simulink model "BANSHEE"  (Simulink 8.7)
settings: Solver=ode1  StartTime=0.0  StopTime=inf  FixedStep=Ts  MaxStep=1e-3  RelTol=1e-3
PostLoadFcn:
  | BANSHEE_init;
InitFcn:
  | BANSHEE_init;
values from neighbouring files (symbols this model uses):
  Ts = 100E-6    (= 0.0001)    [BANSHEE_init.m]
undefined symbols (not defined in the file or in its folder): Acid, Banshee_HWCtrl_IOs, Banshee_SEL751_Woodward_lib, DMS_slave_lib, DMSCommands, F1, F2, F3, fdesignblkfcn, Feeder1_lib, Feeder2_lib, Feeder3_lib, gcbh, generic_ethernet_cb, Lead, Left, relay_housing_lib, SM_UtilityService, SS_F1_RELAY_HOUSING, SS_F2_RELAY_HOUSING, SS_F3_RELAY_HOUSING, SS_Feeder1, SS_Feeder2, SS_Feeder3, SUBSTATION, TestSeq_slave_lib, TestSequenceCommands, type, utility_service_lib, V
libraries: powerlib x108, cables_lib x61, breaker_lib x53, rtio_generic_modbus x50, relay_modbus_lib x45, rtio_opalrt_op5142ex1 x37, transformer_lib x29, rteventslib x28, Load_lib x25, simulink x24, rtlab x20, ssn_lib x19
(part 5 of 9)

== system BANSHEE/SS_F3_RELAY_HOUSING/Banshee UDP Data - Formatted Packets ==
  note: The Number of data to send should match the size of Mux-to-Ethernet
  note: Copyright (c) 2016 Massachusetts Institute of Technology
      | Permission is hereby granted, free of charge, to any person obtaining a copy of this software and associated documentation files (the "Software"), to deal
      | in the Software without restriction, including without limitation the rights to use, copy, modify, merge, publish, distribute, sublicense, and/or sell copies of the
      | Software, and to permit persons to whom the Software is furnished to do so, subject to the following conditions:
      |
      | THE SOFTWARE IS PROVIDED "AS IS", WITHOUT WARRANTY OF ANY KIND, EXPRESS OR IMPLIED, INCLUDING BUT NOT LIMITED TO THE
      | WARRANTIES OF MERCHANTABILITY, FITNESS FOR A PARTICULAR PURPOSE AND NONINFRINGEMENT. IN NO EVENT SHALL THE AUTHORS
      | OR COPYRIGHT HOLDERS BE LIABLE FOR ANY CLAIM, DAMAGES OR OTHER LIABILITY, WHETHER IN AN ACTION OF CONTRACT, TORT OR
      | OTHERWISE, ARISING FROM, OUT OF OR IN CONNECTION WITH THE SOFTWARE OR THE USE OR OTHER DEALINGS IN THE SOFTWARE
  Time Stamp : Inport
  Waveforms : Inport  Port=2  PortDimensions=3
  Relay Data : Inport  Port=3
  BESS Data : Inport  Port=4
  Diesel Gensets Data : Inport  Port=5
  NGCHP Gensets Data : Inport  Port=6
  Motors Data : Inport  Port=7
  PV Data : Inport  Port=8
  Power Factor Data : Inport  Port=9
  Miscellaneous Data : Inport  Port=10
  " # of motors" : Constant  Value=NumOfMotors  OutDataTypeStr=double
  " # of motors1" : Constant  Value=NumOfMiscellaneousDataScales  OutDataTypeStr=double
  # of Batteries : Constant  Value=NumOfBatteries  OutDataTypeStr=double
  # of PVs : Constant  Value=NumOfPVs  OutDataTypeStr=double
  # of PVs1 : Constant  Value=NumOfMiscellaneousDataSignalsScales  OutDataTypeStr=double
  # of PVs2 : Constant  Value=NumOfPF  OutDataTypeStr=double
  # of Relays : Constant  Value=NumOfRelays  OutDataTypeStr=double
  # of Waveform s : Constant  Value=NumOfWaveforms  OutDataTypeStr=double
  # of gensets : Constant  Value=NumOfDieselGensets  OutDataTypeStr=double
  # of gensets1 : Constant  Value=NumOfNGCHPGensets  OutDataTypeStr=double
  Cast uint16 : MATLAB Function  TreatAsAtomicUnit=on
  Checksum : Sum  Inputs=+
  Data Type Conversion : DataTypeConversion
  Data Type Conversion1 : DataTypeConversion  OutDataTypeStr=uint32  ConvertRealWorld=Stored Integer (SI)  RndMeth=Nearest
  Ethernet communication interface : Subsystem  mask(AsyncEthernet){ctrl_id=1, nbr_to_remote_endpoint=375, type_to_remote_endpoint=INT32, offset_to_remote_endpoint=0, swap_tx=off, nbr_from_remote_endpoint=4, type_from_remote_endpoint=DOUBLE, offset_from_remote_endpoint=0, swap_rx=off, exe_name='AsyncEthernet', nic_name='eth0', protocol=UDP, tcp_mode=Server, port=7200, remote_ip='255.255.255.255'}
      mask prompts: ctrl_id "Controller ID"; nbr_to_remote_endpoint "Number of data to send"; type_to_remote_endpoint "Type of data to send"; offset_to_remote_endpoint "Byte offset of transmission buffer"; swap_tx "Swap data endianness before transmission"; nbr_from_remote_endpoint "Number of data expected to be received"; type_from_remote_endpoint "Type of data expected to be received"; offset_from_remote_endpoint "Byte offset of reception buffer"; swap_rx "Swap data endianness after reception"; exe_name "Executable name"; nic_name "Network interface name"; tcp_mode "TCP mode"; port "Port number"; remote_ip "Remote IP address"
      mask help: This block is used as a communication interface to send data to a remote dedevice and receive data from it.
      mask Help: eval('rtlab_io_help(''Generic/Ethernet/Ethernet_interface.htm'');');
      mask Callback ctrl_id:
      | var = get_param(gcb,'ctrl_id');
      | set_param([gcb '/AsyncEthernetCtrl'],'ctrl_id',var)
      mask Callback nbr_to_remote_endpoint:
      | var = get_param(gcb,'nbr_to_remote_endpoint');
      | set_param([gcb '/AsyncEthernetCtrl'],'nbr_to_remote_endpoint',var)
      mask TypeOptions type_to_remote_endpoint: UINT8 | INT8 | UINT16 | INT16 | UINT32 | INT32 | FLOAT | DOUBLE
      mask Callback type_to_remote_endpoint:
      | var = get_param(gcb,'type_to_remote_endpoint');
      | set_param([gcb '/AsyncEthernetCtrl'],'type_to_remote_endpoint',var)
      mask Callback offset_to_remote_endpoint:
      | var = get_param(gcb,'offset_to_remote_endpoint');
      | set_param([gcb '/AsyncEthernetCtrl'],'offset_to_remote_endpoint',var)
      mask Callback swap_tx:
      | var = get_param(gcb,'swap_tx');
      | set_param([gcb '/AsyncEthernetCtrl'],'swap_tx',var)
      mask Callback nbr_from_remote_endpoint:
      | var = get_param(gcb,'nbr_from_remote_endpoint');
      | set_param([gcb '/AsyncEthernetCtrl'],'nbr_from_remote_endpoint',var)
      mask TypeOptions type_from_remote_endpoint: UINT8 | INT8 | UINT16 | INT16 | UINT32 | INT32 | FLOAT | DOUBLE
      mask Callback type_from_remote_endpoint:
      | var = get_param(gcb,'type_from_remote_endpoint');
      | set_param([gcb '/AsyncEthernetCtrl'],'type_from_remote_endpoint',var)
      mask Callback offset_from_remote_endpoint:
      | var = get_param(gcb,'offset_from_remote_endpoint');
      | set_param([gcb '/AsyncEthernetCtrl'],'offset_from_remote_endpoint',var)
      mask Callback swap_rx:
      | var = get_param(gcb,'swap_rx');
      | set_param([gcb '/AsyncEthernetCtrl'],'swap_rx',var)
      mask Callback exe_name:
      | str = get_param(gcb,'exe_name');
      | 
      | if exist('str','var')
      |     str = eval(str);
      | end
      | 
      | set_param([gcb '/AsyncEthernetCtrl'],'exe_name',str)
      mask Callback nic_name:
      | str = get_param(gcb,'nic_name');
      | 
      | if exist('str','var')
      |     str = eval(str);
      | end
      | 
      | set_param([gcb '/AsyncEthernetCtrl'],'nic_name',str)
      mask TypeOptions protocol: UDP | TCP
      mask Callback protocol: generic_ethernet_cb('protocol')
      mask TypeOptions tcp_mode: Client | Server
      mask Callback tcp_mode: generic_ethernet_cb('tcp_mode')
      mask Callback port:
      | var = get_param(gcb,'port');
      | set_param([gcb '/AsyncEthernetCtrl'],'port',var)
      mask Callback remote_ip:
      | str = get_param(gcb,'remote_ip');
      | 
      | if exist('str','var')
      |     str = eval(str);
      | end
      | 
      | set_param([gcb '/AsyncEthernetCtrl'],'remote_ip',str)
  Mux-to-Ethernet : Mux  Inputs=2
  Mux1 : Mux  Inputs=14
  Mux8 : Mux  Inputs=10
  Profile ID : Constant  Value=ProfileID  OutDataTypeStr=double
  Pulse input : DiscretePulseGenerator  PulseType=Time based  Period=1/5  PulseWidth=1/20
  Start Word 0xAFAF : Constant  Value=44975  OutDataTypeStr=double
  Stop Word 0x5555 : Constant  Value=21845  OutDataTypeStr=double
  wires:
  Start Word 0xAFAF/1 -> Mux1/1
  Pulse input/1 -> Data Type Conversion/1
  Data Type Conversion/1 -> Ethernet communication interface/1(Data trigger)
  Mux1/1 -> Mux8/1
  Checksum/1 -> Cast uint16/1(u)
  Cast uint16/1(y) -> Mux-to-Ethernet/2
  Mux-to-Ethernet/1 -> Ethernet communication interface/2(Data to send)
  Data Type Conversion1/1 -> Checksum/1
  Waveforms/1 -> Mux1/14
  BESS Data/1 -> Mux8/3
  Diesel Gensets Data/1 -> Mux8/4
  Relay Data/1 -> Mux8/2
  Mux8/1 -> Mux-to-Ethernet/1, Data Type Conversion1/1
  Stop Word 0x5555/1 -> Mux8/10
  NGCHP Gensets Data/1 -> Mux8/5
  Miscellaneous Data/1 -> Mux8/9
  Power Factor Data/1 -> Mux8/8
  PV Data/1 -> Mux8/7
  Motors Data/1 -> Mux8/6
  Time Stamp/1 -> Mux1/3
  # of PVs1/1 -> Mux1/13
  " # of motors1"/1 -> Mux1/12
  # of gensets1/1 -> Mux1/8
  # of gensets/1 -> Mux1/7
  # of Waveform s/1 -> Mux1/4
  " # of motors"/1 -> Mux1/9
  # of Batteries/1 -> Mux1/6
  # of PVs/1 -> Mux1/10
  # of PVs2/1 -> Mux1/11
  # of Relays/1 -> Mux1/5
  Profile ID/1 -> Mux1/2

== system BANSHEE/SS_F3_RELAY_HOUSING/DMSCommands ==
  note: Copyright (c) 2016 Massachusetts Institute of Technology
      | Permission is hereby granted, free of charge, to any person obtaining a copy of this software and associated documentation files (the "Software"), to deal
      | in the Software without restriction, including without limitation the rights to use, copy, modify, merge, publish, distribute, sublicense, and/or sell copies of the
      | Software, and to permit persons to whom the Software is furnished to do so, subject to the following conditions:
      |
      | THE SOFTWARE IS PROVIDED "AS IS", WITHOUT WARRANTY OF ANY KIND, EXPRESS OR IMPLIED, INCLUDING BUT NOT LIMITED TO THE
      | WARRANTIES OF MERCHANTABILITY, FITNESS FOR A PARTICULAR PURPOSE AND NONINFRINGEMENT. IN NO EVENT SHALL THE AUTHORS
      | OR COPYRIGHT HOLDERS BE LIABLE FOR ANY CLAIM, DAMAGES OR OTHER LIABILITY, WHETHER IN AN ACTION OF CONTRACT, TORT OR
      | OTHERWISE, ARISING FROM, OUT OF OR IN CONNECTION WITH THE SOFTWARE OR THE USE OR OTHER DEALINGS IN THE SOFTWARE
  Add : Sum
  Bus Creator : BusCreator  Inputs=11
  Demux : Demux  Outputs=14
  Gain : Gain  Gain=2^16
  Modbus device : rtio_generic_modbus/Modbus device  conf_name=DMS_cfg.opal  conf_name_mask=DMS_cfg.xls  sample_time=Ts
  Terminator : Terminator
  Terminator1 : Terminator
  DMS Data : Outport
  wires:
  Demux/11 -> Bus Creator/8  "VAR Value"
  Demux/10 -> Bus Creator/7  "VAR Active"
  Demux/9 -> Bus Creator/6  "PF Value"
  Demux/8 -> Bus Creator/5  "PF Active"
  Demux/3 -> Terminator1/1  "Fault1"
  Demux/4 -> Terminator/1  "Fault2"
  Demux/7 -> Bus Creator/4  "Limit Value"
  Demux/6 -> Bus Creator/3  "Limit Active"
  Demux/5 -> Bus Creator/2  "Disconnect"
  Modbus device/1 -> Demux/1
  Gain/1 -> Add/2
  Demux/2 -> Gain/1
  Demux/1 -> Add/1
  Add/1 -> Bus Creator/1  "TimeStamp"
  Bus Creator/1 -> DMS Data/1
  Demux/13 -> Bus Creator/10  "MGC_start"
  Demux/12 -> Bus Creator/9  "AutoSync_available"
  Demux/14 -> Bus Creator/11  "BlackStart"

== system BANSHEE/SS_F3_RELAY_HOUSING/SEL751-UDP ==
  note: Order of signals:
      | F3_PCC
      | F2_PCC
      | F1_PCC
      | F3_GCB (NG/CHP)
      | F1_GCB (DIESEL)
  note: % Copyright (c) 2016 Massachusetts Institute of Technology
      | % Permission is hereby granted, free of charge, to any person obtaining a copy of this
      | % software and associated documentation files (the "Software"), to deal in the Software
      | % without restriction, including without limitation the rights to use, copy, modify,
      | % merge, publish, distribute, sublicense, and/or sell copies of the Software, and to
      | % permit persons to whom the Software is furnished to do so, subject to the following
      | % conditions:
      | %
      | %
      | % The above copyright notice and this permission notice shall be included in
      | % all copies or substantial portions of the Software.
      | %
      | % THE SOFTWARE IS PROVIDED "AS IS", WITHOUT WARRANTY OF ANY KIND, EXPRESS OR IMPLIED,
      | % INCLUDING BUT NOT LIMITED TO THE WARRANTIES OF MERCHANTABILITY, FITNESS FOR A
      | % PARTICULAR PURPOSE AND NONINFRINGEMENT. IN NO EVENT SHALL THE AUTHORS OR COPYRIGHT
      | % HOLDERS BE LIABLE FOR ANY CLAIM, DAMAGES OR OTHER LIABILITY, WHETHER IN AN ACTION
      | % OF CONTRACT, TORT OR OTHERWISE, ARISING FROM, OUT OF OR IN CONNECTION WITH THE
      | % SOFTWARE OR THE USE OR OTHER DEALINGS IN THE SOFTWARE.
      | %
      | %
      | %%
  F3_MS : Inport
  F2_MS : Inport  Port=2
  F1_MS : Inport  Port=3
  Bus Creator : BusCreator  Inputs=5
  Bus Selector : BusSelector  OutputSignals=CB_DATA.F3_PCC
  Bus Selector3 : BusSelector  OutputSignals=CB_DATA.F2_PCC
  Bus Selector5 : BusSelector  OutputSignals=CB_DATA.F1_PCC
  PQFV : PQFV_lib/PQFV  VRMSLL=13800  Ts=Ts
  PQFV1 : PQFV_lib/PQFV  VRMSLL=13800  Ts=Ts
  PQFV2 : PQFV_lib/PQFV  VRMSLL=13800  Ts=Ts
  PQVF_out : Outport
  wires:
  Bus Selector/1 -> PQFV/1  "<F3_PCC>"
  Bus Selector3/1 -> PQFV1/1  "<F2_PCC>"
  F2_MS/1 -> Bus Selector3/1
  Bus Selector5/1 -> PQFV2/1  "<F1_PCC>"
  PQFV1/1 -> Bus Creator/2  "F2_PCC"
  PQFV/1 -> Bus Creator/1  "F3_PCC"
  PQFV2/1 -> Bus Creator/3  "F1_PCC"
  F3_MS/1 -> Bus Creator/4, Bus Selector/1  "F3_MS"
  F1_MS/1 -> Bus Creator/5, Bus Selector5/1  "F1_MS"
  Bus Creator/1 -> PQVF_out/1

== system BANSHEE/SS_Feeder1/fault_signal ==
  fault_ts : Inport
  fault_sc : Inport  Port=2
  Bus Selector26 : BusSelector  OutputSignals=fault_location_2
  Bus Selector28 : BusSelector  OutputSignals=fault_location_2
  Logical Operator : Logic  Operator=OR  AllPortsSameDT=off  OutDataTypeStr=boolean
  o : Outport
  wires:
  fault_sc/1 -> Bus Selector26/1
  Bus Selector26/1 -> Logical Operator/2  "<fault_location_2>"
  fault_ts/1 -> Bus Selector28/1
  Logical Operator/1 -> o/1
  Bus Selector28/1 -> Logical Operator/1  "<fault_location_2>"

== system BANSHEE/SS_Feeder1/fault_signal1 ==
  fault_ts : Inport
  fault_sc : Inport  Port=2
  Bus Selector26 : BusSelector  OutputSignals=fault_location_3
  Bus Selector28 : BusSelector  OutputSignals=fault_location_3
  Logical Operator : Logic  Operator=OR  AllPortsSameDT=off  OutDataTypeStr=boolean
  o : Outport
  wires:
  fault_sc/1 -> Bus Selector26/1
  Bus Selector26/1 -> Logical Operator/2  "<fault_location_3>"
  fault_ts/1 -> Bus Selector28/1
  Logical Operator/1 -> o/1
  Bus Selector28/1 -> Logical Operator/1  "<fault_location_3>"

== system BANSHEE/SS_Feeder2/fault_signal ==
  fault_ts : Inport
  fault_sc : Inport  Port=2
  Bus Selector26 : BusSelector  OutputSignals=fault_location_5
  Bus Selector28 : BusSelector  OutputSignals=fault_location_5
  Logical Operator : Logic  Operator=OR  AllPortsSameDT=off  OutDataTypeStr=boolean
  o : Outport
  wires:
  fault_sc/1 -> Bus Selector26/1
  Bus Selector26/1 -> Logical Operator/2  "<fault_location_5>"
  fault_ts/1 -> Bus Selector28/1
  Logical Operator/1 -> o/1
  Bus Selector28/1 -> Logical Operator/1  "<fault_location_5>"

== system BANSHEE/SS_Feeder2/fault_signal1 ==
  fault_ts : Inport
  fault_sc : Inport  Port=2
  Bus Selector26 : BusSelector  OutputSignals=fault_location_1
  Bus Selector28 : BusSelector  OutputSignals=fault_location_1
  Logical Operator : Logic  Operator=OR  AllPortsSameDT=off  OutDataTypeStr=boolean
  o : Outport
  wires:
  fault_sc/1 -> Bus Selector26/1
  Bus Selector26/1 -> Logical Operator/2  "<fault_location_1>"
  fault_ts/1 -> Bus Selector28/1
  Logical Operator/1 -> o/1
  Bus Selector28/1 -> Logical Operator/1  "<fault_location_1>"

== system BANSHEE/SS_Feeder3/HWController_3.5MVA_NGCHP ==
  note: Copyright (c) 2016 Massachusetts Institute of Technology
      | Permission is hereby granted, free of charge, to any person obtaining a copy of this software and associated documentation files (the "Software"), to deal
      | in the Software without restriction, including without limitation the rights to use, copy, modify, merge, publish, distribute, sublicense, and/or sell copies of the
      | Software, and to permit persons to whom the Software is furnished to do so, subject to the following conditions:
      |
      | THE SOFTWARE IS PROVIDED "AS IS", WITHOUT WARRANTY OF ANY KIND, EXPRESS OR IMPLIED, INCLUDING BUT NOT LIMITED TO THE
      | WARRANTIES OF MERCHANTABILITY, FITNESS FOR A PARTICULAR PURPOSE AND NONINFRINGEMENT. IN NO EVENT SHALL THE AUTHORS
      | OR COPYRIGHT HOLDERS BE LIABLE FOR ANY CLAIM, DAMAGES OR OTHER LIABILITY, WHETHER IN AN ACTION OF CONTRACT, TORT OR
      | OTHERWISE, ARISING FROM, OUT OF OR IN CONNECTION WITH THE SOFTWARE OR THE USE OR OTHER DEALINGS IN THE SOFTWARE
  Heat Load MBtu/hrs : Inport
  In2 : Inport  Port=2
  HWControllerBias : Inport  Port=3
  Bus Creator2 : BusCreator  Inputs=6
  Bus Selector6 : BusSelector  OutputSignals=Heat Recovered; MBtu/hr
  Bus Selector7 : BusSelector  OutputSignals=TempActual,HeatFromBoiler MBtu/hr,CHPHeatContribution MBtu/hr,Thermal data.Heat Recovered; MBtu/hr,Thermal data.CO2 lbm/hr,Boiler_Nm^3/hr ,Boiler lbm/hr CO2
  CHPThermalModel : CHP_Model_lib/CHPThermalModel  SIM_HIL=SIM_HIL
  Demux : Demux  Outputs=2
  HWController_NG_Generator : HWController_NGCHP_Genset_3p5MVA_lib/HWController_NG_Generator
  Modbus device : rtio_generic_modbus/Modbus device  conf_name=CHP_slave_cfg.opal  conf_name_mask=CHP_slave_cfg.xls  sample_time=Ts
  Mux1 : Mux  Inputs=7
  A : PMIOPort  Tag=A  Port=1  Side=Right
      settings: AttributesFormatString=A
  B : PMIOPort  Port=2  Side=Right
  C : PMIOPort  Port=3  Side=Right
  Out1 : Outport
  Generator Data : Outport  Port=2
  GCB Control : Outport  Port=3
  wires:
  Bus Selector7/6 -> Mux1/6  "<Boiler_Nm^3/hr >"
  Bus Selector7/7 -> Mux1/7  "<Boiler lbm/hr CO2 >"
  CHPThermalModel/5 -> Bus Creator2/6
  CHPThermalModel/4 -> Bus Creator2/5
  HWControllerBias/1 -> HWController_NG_Generator/1
  HWController_NG_Generator/3 -> [HeatRec_MBtuhr]  "Thermal data"
  Bus Selector7/3 -> Mux1/3  "<CHPHeatContribution MBtu/hr>"
  CHPThermalModel/1 -> Bus Creator2/2  "TempActual"
  Demux/2 -> CHPThermalModel/4
  CHPThermalModel/2 -> Bus Creator2/3
  Bus Selector7/2 -> Mux1/2  "<HeatFromBoiler MBtu/hr>"
  Bus Selector7/5 -> Mux1/5  "<CO2 lbm/hr>"
  Bus Selector7/4 -> Mux1/4  "<Heat Recovered; MBtu/hr>"
  Bus Selector7/1 -> Mux1/1  "<TempActual>"
  Heat Load MBtu/hrs/1 -> CHPThermalModel/2
  Mux1/1 -> Modbus device/4
  Demux/1 -> CHPThermalModel/3
  CHPThermalModel/3 -> Bus Creator2/4
  [HeatRec_MBtuhr] -> Bus Selector6/1, Bus Creator2/1  "Thermal data"
  Modbus device/2 -> Demux/1
  HWController_NG_Generator/1 -> Generator Data/1
  HWController_NG_Generator/2 -> GCB Control/1
  Bus Selector6/1 -> CHPThermalModel/1  "<Heat Recovered; MBtu/hr>"
  Bus Creator2/1 -> Out1/1, Bus Selector7/1  "CHPData"
  In2/1 -> CHPThermalModel/5  "CHP_SIM_Cmds"
  connections:
  HWController_NG_Generator/RConn3 -- C/RConn1
  HWController_NG_Generator/RConn2 -- B/RConn1
  HWController_NG_Generator/RConn1 -- A/RConn1

== system BANSHEE/SS_Feeder3/fault_signal ==
  fault_ts : Inport
  fault_sc : Inport  Port=2
  Bus Selector26 : BusSelector  OutputSignals=fault_location_4
  Bus Selector28 : BusSelector  OutputSignals=fault_location_4
  Logical Operator : Logic  Operator=OR  AllPortsSameDT=off  OutDataTypeStr=boolean
  o : Outport
  wires:
  fault_sc/1 -> Bus Selector26/1
  Bus Selector26/1 -> Logical Operator/2  "<fault_location_4>"
  fault_ts/1 -> Bus Selector28/1
  Logical Operator/1 -> o/1
  Bus Selector28/1 -> Logical Operator/1  "<fault_location_4>"

== system BANSHEE/SS_PV_BESS/BESS Measurements ==
  note: % Copyright (c) 2016 Massachusetts Institute of Technology
      | % Permission is hereby granted, free of charge, to any person obtaining a copy of this
      | % software and associated documentation files (the "Software"), to deal in the Software
      | % without restriction, including without limitation the rights to use, copy, modify,
      | % merge, publish, distribute, sublicense, and/or sell copies of the Software, and to
      | % permit persons to whom the Software is furnished to do so, subject to the following
      | % conditions:
      | %
      | %
      | % The above copyright notice and this permission notice shall be included in
      | % all copies or substantial portions of the Software.
      | %
      | % THE SOFTWARE IS PROVIDED "AS IS", WITHOUT WARRANTY OF ANY KIND, EXPRESS OR IMPLIED,
      | % INCLUDING BUT NOT LIMITED TO THE WARRANTIES OF MERCHANTABILITY, FITNESS FOR A
      | % PARTICULAR PURPOSE AND NONINFRINGEMENT. IN NO EVENT SHALL THE AUTHORS OR COPYRIGHT
      | % HOLDERS BE LIABLE FOR ANY CLAIM, DAMAGES OR OTHER LIABILITY, WHETHER IN AN ACTION
      | % OF CONTRACT, TORT OR OTHERWISE, ARISING FROM, OUT OF OR IN CONNECTION WITH THE
      | % SOFTWARE OR THE USE OR OTHER DEALINGS IN THE SOFTWARE.
      | %
      | %
      | %%
  EPC_MS : Inport
  Bus Selector33 : BusSelector  OutputSignals=BESS.Battery_Meas.SOC (%),BESS.Battery_Meas.Current (A),BESS.Battery_Meas.Voltage (V),BESS.BESS_MX1.cb_ms.Status,BESS.BESS_MX1.VRMSLL,BESS.BESS_MX1.Freq,BESS.BESS_MX1.kw,BESS.BESS_MX1.kvar
  Gain : Gain  Gain=100
  Gain1 : Gain  Gain=100
  Modbus device6 : rtio_generic_modbus/Modbus device  conf_name=EPC_BMS_cfg.opal  conf_name_mask=EPC_BMS_cfg.xls  sample_time=Ts
  Mux : Mux  Inputs=8
  wires:
  Bus Selector33/5 -> Mux/5  "<VRMSLL>"
  Bus Selector33/3 -> Mux/3  "<Voltage (V)>"
  Bus Selector33/2 -> Mux/2  "<Current (A)>"
  Gain/1 -> Mux/1
  EPC_MS/1 -> Bus Selector33/1
  Bus Selector33/8 -> Mux/8  "<kvar>"
  Bus Selector33/4 -> Mux/4  "<Status>"
  Bus Selector33/7 -> Mux/7  "<kw>"
  Bus Selector33/6 -> Gain1/1  "<Freq>"
  Bus Selector33/1 -> Gain/1  "<SOC (%)>"
  Gain1/1 -> Mux/6
  Mux/1 -> Modbus device6/1

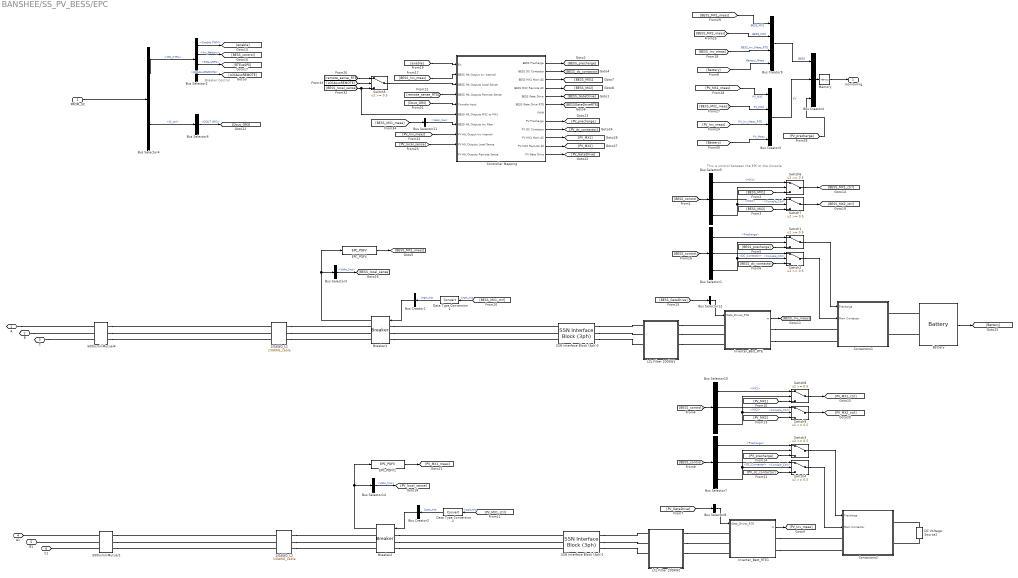
== system BANSHEE/SS_PV_BESS/EPC ==
  note: Breaker Control
  note: This is control between the EPC or the Console
  FROM_SC : Inport
  1/0AWG_L1 : cables_lib/1//0AWG_cable  length=1  par_sets=1
  1/0AWG_L2 : cables_lib/1//0AWG_cable  length=1  par_sets=1
  500kcmil-Mutual1 : cables_lib/500kcmil-Mutual  length=50  par_sets=1  ratio=3
  500kcmil-Mutual4 : cables_lib/500kcmil-Mutual  length=50  par_sets=1  ratio=3
  Battery : electricdrivelib/Extra Sources/Battery  BatType=Lead-Acid  ShowTempParam=off  ThermalPreset=no  NomV=800  NomQ=20000  SOC=80  Batt_Tr=30  PresetModel=on  MaxQ=20833.3333  MinV=600  FullV=871.0526  Dis_rate=4000  R=0.0004  Normal_OP=6205.5556  expZone="[814.4737      66.66667]"  current=[1.5 3]  Units=Ampere-hour  Tci=20  NomT=25  T2=0  MaxQ2=2.208  FullV2=3.45  Normal_OP2=2.8  expZone2="[3.22        0.23]"  Rca=0.6  ti=1000  Dp=0
  Breaker1 : breaker_lib/Breaker  Ts=Ts  mech_delay=0.0833
  Breaker2 : breaker_lib/Breaker  Ts=Ts  mech_delay=0.0833
  Bus Creator1 : BusCreator  Inputs=1
  Bus Creator2 : BusCreator  Inputs=1
  Bus Creator3 : BusCreator  Inputs=4
  Bus Creator4 : BusCreator  Inputs=3
  Bus Creator9 : BusCreator  Inputs=4
  Bus Selector1 : BusSelector  OutputSignals=Precharge,DC_Contactor,Console_Ctrl
  Bus Selector10 : BusSelector  OutputSignals=MX1,MX2,Console_Ctrl
  Bus Selector11 : BusSelector  OutputSignals=cb_ms.Vabc_line
  Bus Selector12 : BusSelector  OutputSignals=signal1,signal2,signal3,signal4,signal5,signal6  OutputAsBus=on
  Bus Selector14 : BusSelector  OutputSignals=Vabc_line
  Bus Selector2 : BusSelector  OutputSignals=Inv_Battery.Enable PWM,Inv_Battery,Inv_Battery.RTEvsSPS,Inv_Battery.LOCALvsREMOTE
  Bus Selector3 : BusSelector  OutputSignals=Vabc_line
  Bus Selector4 : BusSelector  OutputSignals=MN_CTRL,IO_ctrl
  Bus Selector5 : BusSelector  OutputSignals=MX1,MX2,Console_Ctrl
  Bus Selector6 : BusSelector  OutputSignals=DOUT GR3
  Bus Selector7 : BusSelector  OutputSignals=Precharge,DC_Contactor,Console_Ctrl
  Bus Selector8 : BusSelector  OutputSignals=Pulse 1,Pulse 2,Pulse 3,Pulse 4,Pulse 5,Pulse 6  OutputAsBus=on
  Contactors1 : Subsystem
  Contactors2 : Subsystem
  Controller Mapping : Subsystem
  DC Voltage Source2 : powerlib/Electrical Sources/DC Voltage Source  Amplitude=800  Measurements=Voltage
  Data Type Conversion1 : DataTypeConversion
  Data Type Conversion2 : DataTypeConversion
  EPC_PQFV : PQFV_lib/EPC_PQFV  VRMSLL=480  Ts=Ts
  EPC_PQFV1 : PQFV_lib/EPC_PQFV  VRMSLL=480  Ts=Ts
  Inverter_Batt_RTE : Subsystem
  Inverter_Batt_RTE1 : Subsystem
  LCL Filter 200kW1 : Subsystem  mask(LCL Filter){filter_line_ind=50e-6, filter_line_res=0, filter_cap=650e-6, filter_cap_res=100e-3, filter_cap_bleed_res=75e3, filter_inv_ind=85e-6, filter_inv_res=0}
      mask prompts: filter_line_ind "Line Inductor (H)"; filter_line_res "Line Inductor Resistance (Ohm)"; filter_cap "Capacitor (F)"; filter_cap_res "Resistance with Capacitor (ohm)"; filter_cap_bleed_res "Resistance for Capacitor Discharge (ohm)"; filter_inv_ind "Inverter Inductor (H)"; filter_inv_res "Inverter Inductor Resistance (Ohm)"
      mask help: This filter is the LCL filter for the inverter.
  LCL Filter 200kW2 : Subsystem  mask(LCL Filter){filter_line_ind=50e-6, filter_line_res=0, filter_cap=650e-6, filter_cap_res=100e-3, filter_cap_bleed_res=75e3, filter_inv_ind=85e-6, filter_inv_res=0}
      mask prompts: filter_line_ind "Line Inductor (H)"; filter_line_res "Line Inductor Resistance (Ohm)"; filter_cap "Capacitor (F)"; filter_cap_res "Resistance with Capacitor (ohm)"; filter_cap_bleed_res "Resistance for Capacitor Discharge (ohm)"; filter_inv_ind "Inverter Inductor (H)"; filter_inv_res "Inverter Inductor Resistance (Ohm)"
      mask help: This filter is the LCL filter for the inverter.
  Memory : Memory
  SSN Interface Block (3ph)1 : ssn_lib/SSN Interface Block (3ph)  nb_phase=3  nb_port=2  p1_type=V-type(Left)  p2_type=V-type (Right)  p3_type=V-type(Left)  p4_type=V-type(Left)  p5_type=V-type(Left)  p6_type=V-type(Left)  p7_type=V-type(Left)  p8_type=V-type(Left)  p9_type=V-type(Left)  p10_type=V-type(Left)  p11_type=V-type(Left)  p12_type=V-type(Left)  p13_type=V-type(Left)  p14_type=V-type(Left)  p15_type=V-type(Left)  p16_type=V-type(Left)  I_port_shunt_resistance=1e9
  SSN Interface Block (3ph)3 : ssn_lib/SSN Interface Block (3ph)  nb_phase=3  nb_port=2  p1_type=V-type(Left)  p2_type=V-type (Right)  p3_type=V-type(Left)  p4_type=V-type(Left)  p5_type=V-type(Left)  p6_type=V-type(Left)  p7_type=V-type(Left)  p8_type=V-type(Left)  p9_type=V-type(Left)  p10_type=V-type(Left)  p11_type=V-type(Left)  p12_type=V-type(Left)  p13_type=V-type(Left)  p14_type=V-type(Left)  p15_type=V-type(Left)  p16_type=V-type(Left)  I_port_shunt_resistance=1e9
  Switch{1..9} (9 alike) : Switch  Threshold=0.5
  A : PMIOPort  Port=1  Side=Left
  B : PMIOPort  Port=2  Side=Left
  C : PMIOPort  Port=3  Side=Left
  A1 : PMIOPort  Port=4  Side=Left
  B1 : PMIOPort  Port=5  Side=Left
  C1 : PMIOPort  Port=6  Side=Left
  monitoring : Outport
  wires:
  [PV_precharge] -> Bus Creator4/3
  Bus Creator3/1 -> Bus Creator4/2  "PV"
  Bus Creator9/1 -> Bus Creator4/1  "BESS"
  Bus Creator4/1 -> Memory/1
  [Battery] -> Bus Creator3/4  "PV_Meas"
  [PV_MX1_meas] -> Bus Creator3/1  "PV_MX1"
  [BESS_MX2_meas] -> Bus Creator3/2  "PV_MX2"
  [PV_Inv_meas] -> Bus Creator3/3  "PV_Inv_Meas_RTE"
  [PV_local_sense] -> Controller Mapping/9(PV HIL Outputs Local Sense)
  [PV_Inv_meas] -> Controller Mapping/8("PV HIL Output Inv Internal ")
  Controller Mapping/12(PV Gate Drive) -> [PV_GateDrive]
  Controller Mapping/11(PV MX2 Remote AC) -> [PV_MX2]
  Controller Mapping/10(PV MX1 Main AC) -> [PV_MX1]
  Controller Mapping/9(PV DC Contactor) -> [PV_dc_contactor]
  Controller Mapping/8(PV Precharge) -> [PV_precharge]
  Switch9/1 -> [PV_MX2_ctrl]
  Switch8/1 -> [PV_MX1_ctrl]
  [BESS_control] -> Bus Selector10/1
  Bus Selector10/1 -> Switch8/1  "<MX1>"
  Bus Selector10/2 -> Switch9/1  "<MX2>"
  Bus Selector10/3 -> Switch8/2, Switch9/2  "<Console_Ctrl>"
  [PV_MX1] -> Switch8/3
  [PV_MX2] -> Switch9/3
  Bus Selector8/1 -> Inverter_Batt_RTE1/1(Gate_Drives_RTE)
  Bus Selector14/1 -> [PV_local_sense]  "<Vabc_line>"
  EPC_PQFV1/1 -> [PV_MX1_meas]
  [BESS_control] -> Bus Selector7/1
  Inverter_Batt_RTE1/1(m) -> [PV_Inv_meas]
  [PV_GateDrive] -> Bus Selector8/1
  Bus Selector7/1 -> Switch3/1  "<Precharge>"
  Bus Selector7/2 -> Switch4/1  "<DC_Contactor>"
  Bus Selector7/3 -> Switch3/2, Switch4/2  "<Console_Ctrl>"
  Switch3/1 -> Contactors2/1(Precharge)
  Switch4/1 -> Contactors2/2(Main Contactor)
  [PV_precharge] -> Switch3/3
  [PV_dc_contactor] -> Switch4/3
  Switch7/1 -> [BESS_MX2_ctrl]
  Switch6/1 -> [BESS_MX1_ctrl]
  Controller Mapping/4(BESS MX2 Remote AC) -> [BESS_MX2]
  Controller Mapping/3(BESS MX1 Main AC) -> [BESS_MX1]
  [BESS_control] -> Bus Selector5/1
  Bus Selector5/1 -> Switch6/1  "<MX1>"
  Bus Selector5/2 -> Switch7/1  "<MX2>"
  Bus Selector5/3 -> Switch6/2, Switch7/2  "<Console_Ctrl>"
  [BESS_MX1] -> Switch6/3
  [BESS_MX2] -> Switch7/3
  Switch5/1 -> Controller Mapping/3(BESS HIL Outputs Local Sense)
  Bus Selector12/1 -> Inverter_Batt_RTE/1(Gate_Drives_RTE)
  FROM_SC/1 -> Bus Selector4/1
  Bus Selector3/1 -> [BESS_local_sense]  "<Vabc_line>"
  EPC_PQFV/1 -> [BESS_MX1_meas]
  Data Type Conversion1/1 -> Bus Creator1/1  "Logic_trip"
  [Battery] -> Bus Creator9/4  "Battery_Meas"
  [BESS_MX1_meas] -> Bus Creator9/1  "BESS_MX1"
  [BESS_MX2_meas] -> Bus Creator9/2  "BESS_MX2"
  [BESS_Inv_meas] -> Bus Creator9/3  "BESS_Inv_Meas_RTE"
  Bus Selector4/1 -> Bus Selector2/1  "<MN_CTRL>"
  Bus Selector4/2 -> Bus Selector6/1  "<IO_ctrl>"
  Bus Selector6/1 -> [Dout_GR3]  "<DOUT GR3>"
  Bus Selector2/2 -> [BESS_control]  "<Inv_Battery>"
  Bus Selector2/1 -> [enable]  "<Enable PWM>"
  Bus Selector2/3 -> [RTEvsSPS]  "<RTEvsSPS>"
  [remote_sense_RTE] -> Controller Mapping/4(BESS HIL Outputs Remote Sense)
  [Dout_GR3] -> Controller Mapping/5(Console Input)
  Controller Mapping/5(BESS Gate Drive) -> [BESS_GateDrive]
  Controller Mapping/6(BESS Gate Drive RTE) -> [BESSGateDriveRTE]
  [BESS_control] -> Bus Selector1/1
  [enable] -> Controller Mapping/1(En)
  Inverter_Batt_RTE/1(m) -> [BESS_Inv_meas]
  [BESS_Inv_meas] -> Controller Mapping/2("BESS HIL Output Inv Internal ")
  [BESS_GateDrive] -> Bus Selector12/1
  Bus Selector1/1 -> Switch1/1  "<Precharge>"
  Bus Selector1/2 -> Switch2/1  "<DC_Contactor>"
  Bus Selector1/3 -> Switch1/2, Switch2/2  "<Console_Ctrl>"
  Switch1/1 -> Contactors1/1(Precharge)
  Switch2/1 -> Contactors1/2(Main Contactor)
  Bus Selector2/4 -> [LOCALvsREMOTE]  "<LOCALvsREMOTE>"
  [remote_sense_RTE] -> Switch5/1
  [BESS_local_sense] -> Switch5/3, Controller Mapping/6(BESS HIL Outputs MX2 to MX1)
  [LOCALvsREMOTE] -> Switch5/2
  [BESS_MX1_meas] -> Bus Selector11/1
  Bus Selector11/1 -> Controller Mapping/7(BESS HIL Outputs Inv filter)  "<Vabc_line>"
  Controller Mapping/1(BESS Precharge) -> [BESS_precharge]
  [BESS_precharge] -> Switch1/3
  Controller Mapping/2(BESS DC Contactor) -> [BESS_dc_contactor]
  [BESS_dc_contactor] -> Switch2/3
  Memory/1 -> monitoring/1
  Battery/1 -> [Battery]
  [BESS_MX1_ctrl] -> Data Type Conversion1/1  "Logic_trip"
  Bus Creator1/1 -> Breaker1/1
  Breaker1/1 -> EPC_PQFV/1, Bus Selector3/1
  [PV_MX1_ctrl] -> Data Type Conversion2/1  "Logic_trip"
  Bus Creator2/1 -> Breaker2/1
  Data Type Conversion2/1 -> Bus Creator2/1  "Logic_trip"
  Breaker2/1 -> EPC_PQFV1/1, Bus Selector14/1
  connections:
  500kcmil-Mutual1/RConn1 -- 1/0AWG_L2/LConn1
  500kcmil-Mutual1/RConn2 -- 1/0AWG_L2/LConn2
  500kcmil-Mutual1/RConn3 -- 1/0AWG_L2/LConn3
  500kcmil-Mutual4/RConn2 -- 1/0AWG_L1/LConn2
  500kcmil-Mutual4/RConn3 -- 1/0AWG_L1/LConn3
  500kcmil-Mutual4/RConn1 -- 1/0AWG_L1/LConn1
  500kcmil-Mutual1/LConn1 -- A1/RConn1
  500kcmil-Mutual1/LConn2 -- B1/RConn1
  500kcmil-Mutual1/LConn3 -- C1/RConn1
  Inverter_Batt_RTE1/RConn2 -- Contactors2/LConn2
  SSN Interface Block (3ph)1/RConn1 -- LCL Filter 200kW2/LConn1
  Inverter_Batt_RTE1/RConn1 -- Contactors2/LConn1
  SSN Interface Block (3ph)1/RConn2 -- LCL Filter 200kW2/LConn2
  SSN Interface Block (3ph)1/RConn3 -- LCL Filter 200kW2/LConn3
  DC Voltage Source2/RConn1 -- Contactors2/RConn1
  LCL Filter 200kW2/RConn3 -- Inverter_Batt_RTE1/LConn3
  DC Voltage Source2/LConn1 -- Contactors2/RConn2
  LCL Filter 200kW2/RConn2 -- Inverter_Batt_RTE1/LConn2
  LCL Filter 200kW2/RConn1 -- Inverter_Batt_RTE1/LConn1
  LCL Filter 200kW1/RConn1 -- Inverter_Batt_RTE/LConn1
  LCL Filter 200kW1/RConn3 -- Inverter_Batt_RTE/LConn3
  LCL Filter 200kW1/RConn2 -- Inverter_Batt_RTE/LConn2
  Inverter_Batt_RTE/RConn1 -- Contactors1/LConn1
  Inverter_Batt_RTE/RConn2 -- Contactors1/LConn2
  A/RConn1 -- 500kcmil-Mutual4/LConn1
  B/RConn1 -- 500kcmil-Mutual4/LConn2
  C/RConn1 -- 500kcmil-Mutual4/LConn3
  SSN Interface Block (3ph)3/RConn1 -- LCL Filter 200kW1/LConn1
  SSN Interface Block (3ph)3/RConn2 -- LCL Filter 200kW1/LConn2
  SSN Interface Block (3ph)3/RConn3 -- LCL Filter 200kW1/LConn3
  Battery/LConn2 -- Contactors1/RConn2
  Battery/LConn1 -- Contactors1/RConn1
  Breaker1/LConn3 -- SSN Interface Block (3ph)3/LConn3
  Breaker1/LConn2 -- SSN Interface Block (3ph)3/LConn2
  Breaker1/LConn1 -- SSN Interface Block (3ph)3/LConn1
  1/0AWG_L1/RConn3 -- Breaker1/RConn3
  1/0AWG_L1/RConn2 -- Breaker1/RConn2
  1/0AWG_L1/RConn1 -- Breaker1/RConn1
  Breaker2/LConn1 -- SSN Interface Block (3ph)1/LConn1
  Breaker2/LConn3 -- SSN Interface Block (3ph)1/LConn3
  Breaker2/LConn2 -- SSN Interface Block (3ph)1/LConn2
  1/0AWG_L2/RConn2 -- Breaker2/RConn2
  1/0AWG_L2/RConn3 -- Breaker2/RConn3
  1/0AWG_L2/RConn1 -- Breaker2/RConn1

== system BANSHEE/SS_PV_BESS/PV Measurements ==
  note: % Copyright (c) 2016 Massachusetts Institute of Technology
      | % Permission is hereby granted, free of charge, to any person obtaining a copy of this
      | % software and associated documentation files (the "Software"), to deal in the Software
      | % without restriction, including without limitation the rights to use, copy, modify,
      | % merge, publish, distribute, sublicense, and/or sell copies of the Software, and to
      | % permit persons to whom the Software is furnished to do so, subject to the following
      | % conditions:
      | %
      | %
      | % The above copyright notice and this permission notice shall be included in
      | % all copies or substantial portions of the Software.
      | %
      | % THE SOFTWARE IS PROVIDED "AS IS", WITHOUT WARRANTY OF ANY KIND, EXPRESS OR IMPLIED,
      | % INCLUDING BUT NOT LIMITED TO THE WARRANTIES OF MERCHANTABILITY, FITNESS FOR A
      | % PARTICULAR PURPOSE AND NONINFRINGEMENT. IN NO EVENT SHALL THE AUTHORS OR COPYRIGHT
      | % HOLDERS BE LIABLE FOR ANY CLAIM, DAMAGES OR OTHER LIABILITY, WHETHER IN AN ACTION
      | % OF CONTRACT, TORT OR OTHERWISE, ARISING FROM, OUT OF OR IN CONNECTION WITH THE
      | % SOFTWARE OR THE USE OR OTHER DEALINGS IN THE SOFTWARE.
      | %
      | %
      | %%
  EPC_MS : Inport
  Bus Selector33 : BusSelector  OutputSignals=PV.PV_Meas.Current (A),PV.PV_Meas.Voltage (V),PV.PV_MX1.cb_ms.Status,PV.PV_MX1.VRMSLL,PV.PV_MX1.Freq,PV.PV_MX1.kw,PV.PV_MX1.kvar
  Gain1 : Gain  Gain=100
  Modbus device6 : rtio_generic_modbus/Modbus device  conf_name=EPC_PVMS_cfg.opal  conf_name_mask=EPC_PVMS_cfg.xls  sample_time=Ts
  Mux : Mux  Inputs=8
  NA : Constant
  wires:
  EPC_MS/1 -> Bus Selector33/1
  Mux/1 -> Modbus device6/1
  Bus Selector33/5 -> Gain1/1  "<Freq>"
  NA/1 -> Mux/1
  Bus Selector33/4 -> Mux/5  "<VRMSLL>"
  Bus Selector33/3 -> Mux/4  "<Status>"
  Bus Selector33/2 -> Mux/3  "<Voltage (V)>"
  Bus Selector33/1 -> Mux/2  "<Current (A)>"
  Gain1/1 -> Mux/6
  Bus Selector33/7 -> Mux/8  "<kvar>"
  Bus Selector33/6 -> Mux/7  "<kw>"

== system BANSHEE/SC_ctrl/EPC Inverter/16Din/16Dout GR3 ==
  note: Ch12-15
  note: Ch08-11
  note: Ch04-07
  note: Ch00-03
  Din : Inport
  Bus Creator{,1..3,6} (5 alike) : BusCreator  Inputs=4
  Constant{1,3,5,7} (4 alike) : Constant  Value=0
  Constant{2,4,6,8} (4 alike) : Constant
  DO0_Estop : ManualSwitch
  DO10_ExtAlarm : ManualSwitch  CurrentSetting=0
  DO11_EnableMCB : ManualSwitch  CurrentSetting=0
  DO12_MCBOpen : ManualSwitch  CurrentSetting=0
  DO13_GCBOpen : ManualSwitch  CurrentSetting=0
  DO{6..7,14..15} (4 alike) : ManualSwitch  CurrentSetting=0
  DO1_Start/Auto : ManualSwitch  CurrentSetting=0
  DO2_ExtAlarm : ManualSwitch  CurrentSetting=0
  DO3_EnableMCB : ManualSwitch  CurrentSetting=0
  DO4_MCBOpen : ManualSwitch  CurrentSetting=0
  DO5_GCBOpen : ManualSwitch  CurrentSetting=0
  DO8_Estop : ManualSwitch
  DO9_Start/Auto : ManualSwitch  CurrentSetting=0
  Display{,1..15} (16 alike) : Display
  Dout : Outport
  wires:
  ? -> Display7/1  "<Gen1_Alarm_AB>"
  ? -> Display4/1  "<Gen1_Open_GCB>"
  ? -> Display15/1  "<Gen2_Alarm_CF>"
  ? -> Display14/1  "<Gen2_Alarm_AB>"
  ? -> Display13/1  "<Gen2_Open_MCB>"
  ? -> Display12/1  "<Gen2_Close_MCB>"
  ? -> Display11/1  "<Gen2_Open_GCB>"
  ? -> Display10/1  "<Gen2_Close_GCB>"
  ? -> Display9/1  "<Gen2_Fuel>"
  ? -> Display1/1  "<Gen2_Starter>"
  ? -> ?  "<DI_CH08-15>"
  ? -> Display8/1  "<Gen1_Alarm_CF>"
  ? -> Display6/1  "<Gen1_Open_MCB>"
  ? -> Display5/1  "<Gen1_Close_MCB>"
  ? -> Display3/1  "<Gen1_Close_GCB>"
  ? -> Display2/1  "<Gen1_Fuel>"
  ? -> Display/1  "<Gen1_Starter>"
  ? -> ?  "<DI_CH00-07>"
  Din/1 -> ?
  [T3] -> Bus Creator6/4  "12-15"
  [T2] -> Bus Creator6/3  "08-11"
  [T1] -> Bus Creator6/2  "04-07"
  [T0] -> Bus Creator6/1  "00-03"
  Bus Creator2/1 -> [T2]
  Bus Creator3/1 -> [T3]
  Bus Creator1/1 -> [T1]
  Bus Creator/1 -> [T0]
  DO15/1 -> Bus Creator3/4  "Gen2_DI12_GCB_Busbar"
  DO14/1 -> Bus Creator3/3  "Gen2_DI11_MCB_Busbar"
  DO13_GCBOpen/1 -> Bus Creator3/2  "Gen2_GCBOpen"
  DO12_MCBOpen/1 -> Bus Creator3/1  "Gen2_MCBOpen"
  Constant7/1 -> DO12_MCBOpen/2, DO13_GCBOpen/2, DO15/2, DO14/2
  Constant8/1 -> DO12_MCBOpen/1, DO13_GCBOpen/1, DO15/1, DO14/1
  DO11_EnableMCB/1 -> Bus Creator2/4  "Gen2_EnableMCB"
  DO10_ExtAlarm/1 -> Bus Creator2/3  "Gen2_ExtAlarm"
  DO9_Start/Auto/1 -> Bus Creator2/2  "Gen2_StartAuto"
  DO8_Estop/1 -> Bus Creator2/1  "Gen2_Estop"
  Constant5/1 -> DO10_ExtAlarm/2, DO11_EnableMCB/2, DO9_Start/Auto/2, DO8_Estop/2
  Constant6/1 -> DO10_ExtAlarm/1, DO11_EnableMCB/1, DO9_Start/Auto/1, DO8_Estop/1
  DO7/1 -> Bus Creator1/4  "Gen1_DI12_GCB_Busbar"
  DO6/1 -> Bus Creator1/3  "Gen1_DI11_MCB_Busbar"
  DO5_GCBOpen/1 -> Bus Creator1/2  "Gen1_GCBOpen"
  DO4_MCBOpen/1 -> Bus Creator1/1  "Gen1_MCBOpen"
  Constant3/1 -> DO4_MCBOpen/2, DO5_GCBOpen/2, DO7/2, DO6/2
  Constant4/1 -> DO4_MCBOpen/1, DO5_GCBOpen/1, DO7/1, DO6/1
  DO3_EnableMCB/1 -> Bus Creator/4  "Gen1_EnableMCB"
  DO2_ExtAlarm/1 -> Bus Creator/3  "Gen1_ExtAlarm"
  DO1_Start/Auto/1 -> Bus Creator/2  "Gen1_StartAuto"
  DO0_Estop/1 -> Bus Creator/1  "Gen1_Estop"
  Constant1/1 -> DO2_ExtAlarm/2, DO3_EnableMCB/2, DO1_Start/Auto/2, DO0_Estop/2
  Constant2/1 -> DO2_ExtAlarm/1, DO3_EnableMCB/1, DO1_Start/Auto/1, DO0_Estop/1
  Bus Creator6/1 -> Dout/1  "DO"

== system BANSHEE/SC_ctrl/EPC Inverter/16PWMIn/16PWMout GR3 ==
  A17 : Constant  Value=0.1
  A18 : Constant  Value=0.2
  A19 : Constant  Value=0.3
  A20 : Constant  Value=0.4
  A21 : Constant  Value=0.5
  A22 : Constant  Value=0.6
  A23 : Constant  Value=0.7
  A24 : Constant  Value=0.8
  A25 : Constant  Value=0.2
  A26 : Constant  Value=0.3
  A27 : Constant  Value=0.4
  A28 : Constant  Value=0.5
  A29 : Constant  Value=0.6
  A30 : Constant  Value=0.7
  A31 : Constant  Value=0.8
  A32 : Constant  Value=0.1
  B17 : Constant  Value=10000
  B18 : Constant  Value=5500
  B19 : Constant  Value=5000
  B20 : Constant  Value=4500
  B21 : Constant  Value=4000
  B22 : Constant  Value=3500
  B23 : Constant  Value=3000
  B24 : Constant  Value=2500
  B25 : Constant  Value=9500
  B26 : Constant  Value=9000
  B27 : Constant  Value=8500
  B28 : Constant  Value=8000
  B29 : Constant  Value=7500
  B30 : Constant  Value=7000
  B31 : Constant  Value=6500
  B32 : Constant  Value=6000
  Bus Creator{7..8,10..11} (4 alike) : BusCreator  Inputs=8
  Bus Creator12 : BusCreator  Inputs=2
  Bus Creator6 : BusCreator  Inputs=2
  Bus Creator9 : BusCreator  Inputs=2
  To PWMOut : Outport
  wires:
  Bus Creator9/1 -> Bus Creator6/1  "Ch16-23"
  Bus Creator12/1 -> Bus Creator6/2  "Ch24-31"
  Bus Creator11/1 -> Bus Creator12/1  "FreqPWMOut24-31"
  Bus Creator10/1 -> Bus Creator12/2  "DutyPWMOut24-31"
  B24/1 -> Bus Creator11/8  "FreqCh31"
  B23/1 -> Bus Creator11/7  "FreqCh30"
  B22/1 -> Bus Creator11/6  "FreqCh29"
  B21/1 -> Bus Creator11/5  "FreqCh28"
  B20/1 -> Bus Creator11/4  "FreqCh27"
  B19/1 -> Bus Creator11/3  "FreqCh26"
  B18/1 -> Bus Creator11/2  "FreqCh25"
  B32/1 -> Bus Creator11/1  "FreqCh24"
  A24/1 -> Bus Creator10/8  "DutyCh31"
  A23/1 -> Bus Creator10/7  "DutyCh30"
  A22/1 -> Bus Creator10/6  "DutyCh29"
  A21/1 -> Bus Creator10/5  "DutyCh28"
  A20/1 -> Bus Creator10/4  "DutyCh27"
  A19/1 -> Bus Creator10/3  "DutyCh26"
  A18/1 -> Bus Creator10/2  "DutyCh25"
  A32/1 -> Bus Creator10/1  "DutyCh24"
  Bus Creator8/1 -> Bus Creator9/1  "FreqPWMOut16-23"
  Bus Creator7/1 -> Bus Creator9/2  "DutyPWMOut16-23"
  B31/1 -> Bus Creator8/8  "FreqCh23"
  B30/1 -> Bus Creator8/7  "FreqCh22"
  B29/1 -> Bus Creator8/6  "FreqCh21"
  B28/1 -> Bus Creator8/5  "FreqCh20"
  B27/1 -> Bus Creator8/4  "FreqCh19"
  B26/1 -> Bus Creator8/3  "FreqCh18"
  B25/1 -> Bus Creator8/2  "FreqCh17"
  B17/1 -> Bus Creator8/1  "FreqCh16"
  A31/1 -> Bus Creator7/8  "DutyCh23"
  A30/1 -> Bus Creator7/7  "DutyCh22"
  A29/1 -> Bus Creator7/6  "DutyCh21"
  A28/1 -> Bus Creator7/5  "DutyCh20"
  A27/1 -> Bus Creator7/4  "DutyCh19"
  A26/1 -> Bus Creator7/3  "DutyCh18"
  A25/1 -> Bus Creator7/2  "DutyCh17"
  A17/1 -> Bus Creator7/1  "DutyCh16"
  Bus Creator6/1 -> To PWMOut/1

== system BANSHEE/SC_ctrl/EPC Inverter/16TSDIn/16 TSDOut GR3 ==
  Bus Creator1 : BusCreator  Inputs=3
  Din/Dout ch16-23 : Subsystem
  Din/Dout ch24-31 : Subsystem
  Dout state ctrl : Subsystem
  TSDout : Outport
  wires:
  Bus Creator1/1 -> TSDout/1
  Dout state ctrl/1(Event State OUT) -> Bus Creator1/3  "states"
  Din/Dout ch16-23/1(Out1) -> Bus Creator1/1  "times CH16-23"
  Din/Dout ch24-31/1(Out1) -> Bus Creator1/2  "times CH24-31"

== system BANSHEE/SC_ctrl/Woodward/16Din/16Dout GR3 ==
  note: Ch00-03
  note: Ch04-07
  note: Ch08-11
  note: Ch12-15
  note: Enable
  note: Reset
  Bus Creator{,1..3} (4 alike) : BusCreator  Inputs=4
  Bus Creator4 : BusCreator  Inputs=3
  Bus Creator6 : BusCreator  Inputs=5
  CHP Enable/Disable : ManualSwitch  CurrentSetting=0
  CHP Reset : ManualSwitch  CurrentSetting=0
  CHP TempSetPoint : Constant  Value=20.05
  Constant{1,3,5,7} (4 alike) : Constant  Value=0
  Constant{2,4,6,8} (4 alike) : Constant
  DO0_Estop : ManualSwitch
  DO10_ExtAlarm : ManualSwitch  CurrentSetting=0
  DO11_EnableMCB : ManualSwitch  CurrentSetting=0
  DO12_MCBOpen : ManualSwitch  CurrentSetting=0
  DO13_GCBOpen : ManualSwitch  CurrentSetting=0
  DO{6..7,14..15} (4 alike) : ManualSwitch  CurrentSetting=0
  DO1_Start/Auto : ManualSwitch  CurrentSetting=0
  DO2_ExtAlarm : ManualSwitch  CurrentSetting=0
  DO3_EnableMCB : ManualSwitch  CurrentSetting=0
  DO4_MCBClose : ManualSwitch
  DO5_GCBClose : ManualSwitch
  DO8_Estop : ManualSwitch
  DO9_Start/Auto : ManualSwitch  CurrentSetting=0
  Dout : Outport
  wires:
  Bus Creator4/1 -> Bus Creator6/5  "CHP_SIM_Cmds"
  CHP Reset/1 -> Bus Creator4/3  "CHP Reset"
  CHP TempSetPoint/1 -> Bus Creator4/2  "CHP TempSetPoint"
  CHP Enable/Disable/1 -> Bus Creator4/1  "CHP Enable/Disable"
  Bus Creator6/1 -> Dout/1  "DO"
  Constant2/1 -> DO0_Estop/1, DO1_Start/Auto/1, DO3_EnableMCB/1, DO2_ExtAlarm/1
  Constant1/1 -> DO0_Estop/2, DO1_Start/Auto/2, DO3_EnableMCB/2, DO2_ExtAlarm/2
  DO0_Estop/1 -> Bus Creator/1  "Gen1_Estop"
  DO1_Start/Auto/1 -> Bus Creator/2  "Gen1_StartAuto"
  DO2_ExtAlarm/1 -> Bus Creator/3  "Gen1_ExtAlarm"
  DO3_EnableMCB/1 -> Bus Creator/4  "Gen1_EnableMCB"
  Constant4/1 -> DO6/1, DO7/1, CHP Enable/Disable/1, CHP Reset/1, DO5_GCBClose/1, DO4_MCBClose/1
  Constant3/1 -> DO6/2, CHP Enable/Disable/2, CHP Reset/2, DO7/2, DO5_GCBClose/2, DO4_MCBClose/2
  DO4_MCBClose/1 -> Bus Creator1/1  "Gen1_MCBOpen"
  DO5_GCBClose/1 -> Bus Creator1/2  "Gen1_GCBOpen"
  DO6/1 -> Bus Creator1/3  "Gen1_DI11_MCB_Busbar"
  DO7/1 -> Bus Creator1/4  "Gen1_DI12_GCB_Busbar"
  Constant6/1 -> DO8_Estop/1, DO9_Start/Auto/1, DO11_EnableMCB/1, DO10_ExtAlarm/1
  Constant5/1 -> DO8_Estop/2, DO9_Start/Auto/2, DO11_EnableMCB/2, DO10_ExtAlarm/2
  DO8_Estop/1 -> Bus Creator2/1  "Gen2_Estop"
  DO9_Start/Auto/1 -> Bus Creator2/2  "Gen2_StartAuto"
  DO10_ExtAlarm/1 -> Bus Creator2/3  "Gen2_ExtAlarm"
  DO11_EnableMCB/1 -> Bus Creator2/4  "Gen2_EnableMCB"
  Constant8/1 -> DO14/1, DO15/1, DO13_GCBOpen/1, DO12_MCBOpen/1
  Constant7/1 -> DO14/2, DO15/2, DO13_GCBOpen/2, DO12_MCBOpen/2
  DO12_MCBOpen/1 -> Bus Creator3/1  "Gen2_MCBOpen"
  DO13_GCBOpen/1 -> Bus Creator3/2  "Gen2_GCBOpen"
  DO14/1 -> Bus Creator3/3  "Gen2_DI11_MCB_Busbar"
  DO15/1 -> Bus Creator3/4  "Gen2_DI12_GCB_Busbar"
  Bus Creator/1 -> [T0]
  Bus Creator1/1 -> [T1]
  Bus Creator3/1 -> [T3]
  Bus Creator2/1 -> [T2]
  [T0] -> Bus Creator6/1  "00-03"
  [T1] -> Bus Creator6/2  "04-07"
  [T2] -> Bus Creator6/3  "08-11"
  [T3] -> Bus Creator6/4  "12-15"

== system BANSHEE/SM_UtilityService/Banshee_HWCtrl_IOs/GR1 B AIN (CH00-15) ==
  AnalogIn : rtio_opalrt_common/AnalogIn  CtrlName='OpCtrl'  portNb=1  FcnNos=Slot 1 Module B Subsection 1  size=16  maxcount=8  count=8  numchan=8  sampleTime=0
      settings: AttributesFormatString=%<CtrlName>
  AnalogIn1 : rtio_opalrt_common/AnalogIn  CtrlName='OpCtrl'  portNb=2  FcnNos=Slot 1 Module B Subsection 2  size=16  maxcount=8  count=8  numchan=8  sampleTime=0
      settings: AttributesFormatString=%<CtrlName>
  Mux6 : Mux  Inputs=2
  Terminator2 : Terminator
  Terminator3 : Terminator
  Out1 : Outport
  wires:
  Mux6/1 -> Out1/1
  AnalogIn1/2 -> Terminator3/1
  AnalogIn/2 -> Terminator2/1
  AnalogIn1/1 -> Mux6/2
  AnalogIn/1 -> Mux6/1
